simulink model "task4_lab12"  (R2021a)
settings: Solver=VariableStepAuto  StartTime=0.0  StopTime=10.0  RelTol=1e-3
libraries: simulink x1
settings Model: Creator=reemb  LastModifiedBy=reemb

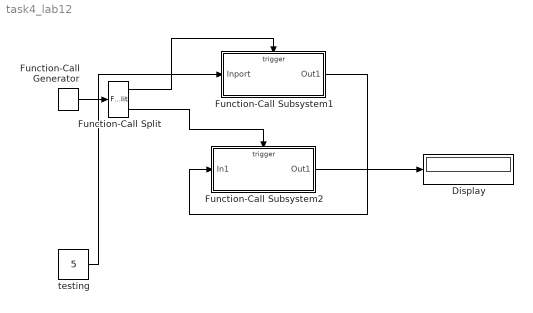
== system task4_lab12 ==
  Display : Display
  Function-Call Generator : simulink/Ports & Subsystems/Function-Call Generator  sample_time=1  numberOfIterations=1  DisallowWideOutput=off
  Function-Call Split : FunctionCallSplit  IconShape=distinctive  NumOutputPorts=2  OutputPortLayout=default
  Function-Call Subsystem1 : Subsystem  TreatAsAtomicUnit=on
  Function-Call Subsystem2 : Subsystem  TreatAsAtomicUnit=on
  testing : Constant  Value=5
  wires:
  Function-Call Generator/1 -> Function-Call Split/1
  Function-Call Split/1 -> Function-Call Subsystem1/Trigger
  Function-Call Split/2 -> Function-Call Subsystem2/Trigger
  Function-Call Subsystem1/1(Out1) -> Function-Call Subsystem2/1(In1)
  testing/1 -> Function-Call Subsystem1/1(Inport)
  Function-Call Subsystem2/1(Out1) -> Display/1

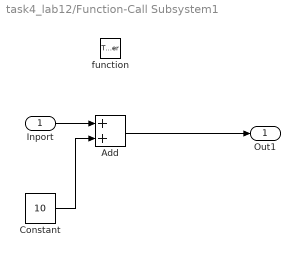
== system task4_lab12/Function-Call Subsystem1 ==
  Inport : Inport
  function : TriggerPort  TriggerType=function-call  VariantControl=(inherit)
  Add : Sum
  Constant : Constant  Value=10
  Out1 : Outport
  wires:
  Constant/1 -> Add/2
  Add/1 -> Out1/1
  Inport/1 -> Add/1

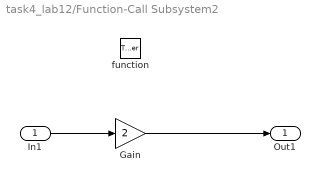
== system task4_lab12/Function-Call Subsystem2 ==
  In1 : Inport
  function : TriggerPort  TriggerType=function-call  VariantControl=(inherit)
  Gain : Gain  Gain=2
  Out1 : Outport
  wires:
  In1/1 -> Gain/1
  Gain/1 -> Out1/1
